simulink model "bankAngleXtkTae"  (R2020b)
settings: Solver=VariableStepAuto  StartTime=0.0  StopTime=80  RelTol=1e-3
values from neighbouring files (symbols this model uses):
  K = place(sys.A,sys.B,p)    [identification.m]
  sys = ssest(data,nx)    [identification.m]
settings Model: Creator=florian  LastModifiedBy=florian

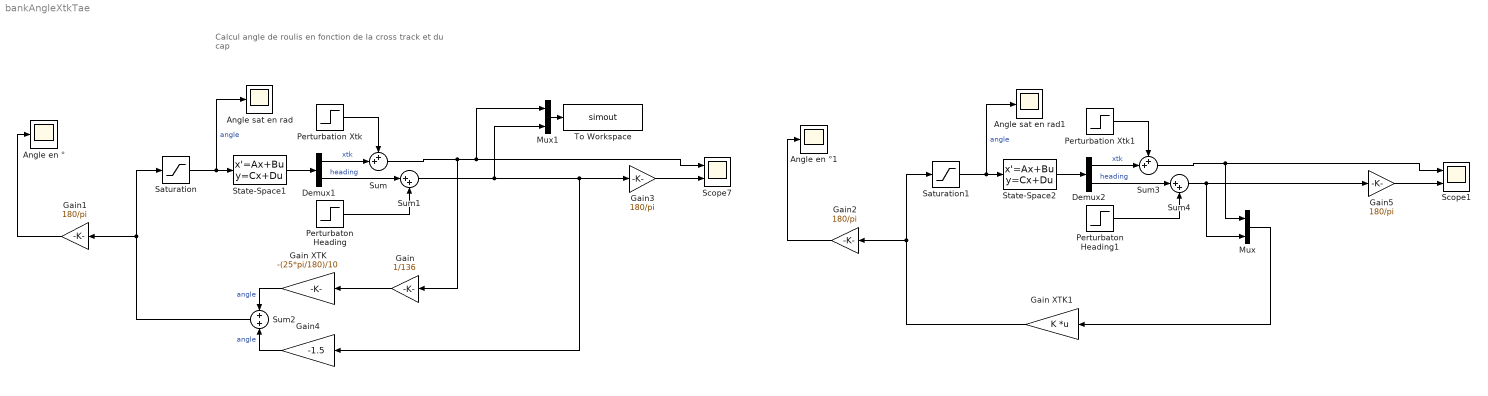
== system bankAngleXtkTae ==
  note: Calcul angle de roulis en fonction de la cross track et du cap
  Angle en ° : Scope
  Angle en °1 : Scope
  Angle sat en rad : Scope
  Angle sat en rad1 : Scope
  Demux1 : Demux  Outputs=2
  Demux2 : Demux  Outputs=2
  Gain : Gain  Gain=1/136
  Gain XTK : Gain  Gain=-(25*pi/180)/10
  Gain XTK1 : Gain  Gain=K  Multiplication=Matrix(K*u)
  Gain{1..3,5} (4 alike) : Gain  Gain=180/pi
  Gain4 : Gain  Gain=-1.5
  Mux : Mux  Inputs=2
  Mux1 : Mux  Inputs=2
  Perturbation Xtk : Step  After=10  SampleTime=0
  Perturbation Xtk1 : Step  After=10  SampleTime=0
  Perturbaton Heading : Step  Time=2  After=0  SampleTime=0
  Perturbaton Heading1 : Step  Time=2  After=0  SampleTime=0
  Saturation : Saturate  UpperLimit=25*pi/180  LowerLimit=-25*pi/180
  Saturation1 : Saturate  UpperLimit=25*pi/180  LowerLimit=-25*pi/180
  Scope1 : Scope  NumInputPorts=2
  Scope7 : Scope  NumInputPorts=2
  State-Space1 : StateSpace  A=sys.A  B=sys.B  C=sys.C  D=sys.D  InitialCondition=0
  State-Space2 : StateSpace  A=sys.A  B=sys.B  C=sys.C  D=sys.D  InitialCondition=0
  Sum : Sum  Inputs=++|
  Sum1 : Sum  Inputs=|++
  Sum2 : Sum
  Sum3 : Sum  Inputs=++|
  Sum4 : Sum  Inputs=|++
  To Workspace : ToWorkspace  VariableName=simout  SaveFormat=Structure With Time  SampleTime=-1
  wires:
  Sum/1 -> Gain/1, Mux1/1, Scope7/1
  Demux1/1 -> Sum/2  "xtk"
  Perturbation Xtk/1 -> Sum/1
  Perturbaton Heading/1 -> Sum1/2
  State-Space1/1 -> Demux1/1
  Demux1/2 -> Sum1/1  "heading"
  Sum1/1 -> Mux1/2, Gain4/1, Gain3/1
  Gain1/1 -> Angle en °/1
  Saturation/1 -> Angle sat en rad/1, State-Space1/1  "angle"
  Gain3/1 -> Scope7/2
  Gain XTK/1 -> Sum2/1  "angle"
  Sum2/1 -> Saturation/1, Gain1/1
  Gain4/1 -> Sum2/2  "angle"
  Perturbaton Heading1/1 -> Sum4/2
  Saturation1/1 -> Angle sat en rad1/1, State-Space2/1  "angle"
  Perturbation Xtk1/1 -> Sum3/1
  Gain5/1 -> Scope1/2
  Demux2/1 -> Sum3/2  "xtk"
  Gain XTK1/1 -> Saturation1/1, Gain2/1
  Sum4/1 -> Mux/2, Gain5/1
  State-Space2/1 -> Demux2/1
  Demux2/2 -> Sum4/1  "heading"
  Sum3/1 -> Mux/1, Scope1/1
  Gain2/1 -> Angle en °1/1
  Mux/1 -> Gain XTK1/1
  Mux1/1 -> To Workspace/1
  Gain/1 -> Gain XTK/1
